simulink model "Robot_Model_Park"  (R2012b)
settings: Solver=ode45  StartTime=0.0  StopTime=T  FixedStep=dt  RelTol=1e-3
values from neighbouring files (symbols this model uses):
  bx = [0; 800; 800; 1600; 1600; 1600+L; 1600+L; 2400+L]    [TrajectoryCalc.m]
  by = [-dwall; -dwall; D-dwall; D-dwall; -dwall; -dwall; D-dwall; D-dwall]    [TrajectoryCalc.m]
  omega_park = [omega_park1; omega_park2; omega_park3]    [TrajectoryCalc.m]
  omegamax = 150*pi/180    (= 2.61799387799)    [TrajectoryCalc.m]
  psi0 = psi_park2(end)    [TrajectoryCalc.m]
  v_park = [v_park1; v_park2; v_park3]    [TrajectoryCalc.m]
  vmax = 500    [TrajectoryCalc.m]
  x0 = px_park2(end)    [TrajectoryCalc.m]
  y0 = py_park2(end)    [TrajectoryCalc.m]
settings Model: Creator=showe023  LastModifiedBy=Daniel
settings DataIOCC: SignalLoggingSaveFormat=ModelDataLogs
settings OptimizationCC: ExpressionDepthLimit=128
settings DebuggingCC: SolverPrmCheckMsg=none  MultiTaskDSMMsg=warning  MultiTaskCondExecSysMsg=none  StrictBusMsg=None
settings RTWCC: IncludeERTFirstTime=on
settings CodeAppCC: CustomSymbolStrType=$N$R$M_T  InternalIdentifier=Shortened

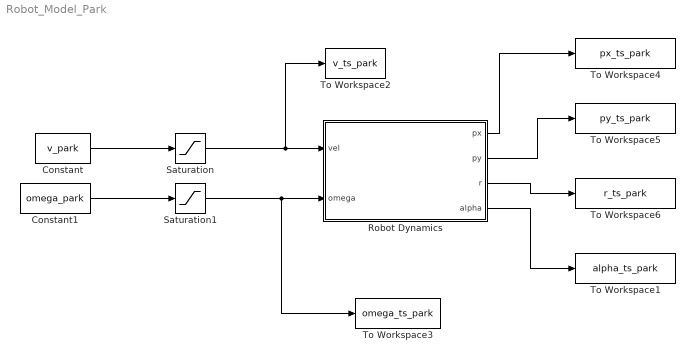
== system Robot_Model_Park ==
  Constant : Constant  Value=v_park
  Constant1 : Constant  Value=omega_park
  Robot Dynamics : Subsystem
  Saturation : Saturate  UpperLimit=vmax  LowerLimit=-vmax
  Saturation1 : Saturate  UpperLimit=omegamax  LowerLimit=-omegamax
  To Workspace1 : ToWorkspace  VariableName=alpha_ts_park  SampleTime=-1  SaveFormat=Timeseries
  To Workspace2 : ToWorkspace  VariableName=v_ts_park  SampleTime=-1  SaveFormat=Timeseries
  To Workspace3 : ToWorkspace  VariableName=omega_ts_park  SampleTime=-1  SaveFormat=Timeseries
  To Workspace4 : ToWorkspace  VariableName=px_ts_park  SampleTime=-1  SaveFormat=Timeseries
  To Workspace5 : ToWorkspace  VariableName=py_ts_park  SampleTime=-1  SaveFormat=Timeseries
  To Workspace6 : ToWorkspace  VariableName=r_ts_park  SampleTime=-1  SaveFormat=Timeseries
  wires:
  Robot Dynamics/1(px) -> To Workspace4/1
  Constant/1 -> Saturation/1
  Saturation/1 -> Robot Dynamics/1(vel), To Workspace2/1
  Robot Dynamics/2(py) -> To Workspace5/1
  Robot Dynamics/3(r) -> To Workspace6/1
  Robot Dynamics/4(alpha) -> To Workspace1/1
  Constant1/1 -> Saturation1/1
  Saturation1/1 -> To Workspace3/1, Robot Dynamics/2(omega)

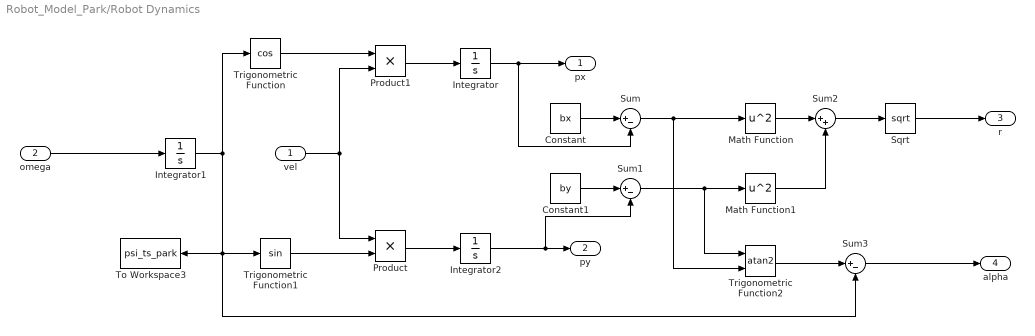
== system Robot_Model_Park/Robot Dynamics ==
  vel : Inport
  omega : Inport  Port=2
  Constant : Constant  Value=bx
  Constant1 : Constant  Value=by
  Integrator : Integrator  InitialCondition=x0
  Integrator1 : Integrator  InitialCondition=psi0
  Integrator2 : Integrator  InitialCondition=y0
  Math Function : Math  Operator=square  SaturateOnIntegerOverflow=on
  Math Function1 : Math  Operator=square  SaturateOnIntegerOverflow=on
  Product : Product
  Product1 : Product
  Sqrt : Sqrt  SaturateOnIntegerOverflow=on
  Sum : Sum  Inputs=|+-
  Sum1 : Sum  Inputs=|+-
  Sum2 : Sum  Inputs=|++
  Sum3 : Sum  Inputs=|+-
  To Workspace3 : ToWorkspace  VariableName=psi_ts_park  SampleTime=-1  SaveFormat=Timeseries
  Trigonometric Function : Trigonometry  Operator=cos
  Trigonometric Function1 : Trigonometry
  Trigonometric Function2 : Trigonometry  Operator=atan2
  px : Outport
  py : Outport  Port=2
  r : Outport  Port=3
  alpha : Outport  Port=4
  wires:
  omega/1 -> Integrator1/1
  Integrator1/1 -> Sum3/2, Trigonometric Function1/1, To Workspace3/1, Trigonometric Function/1
  Trigonometric Function/1 -> Product1/1
  Trigonometric Function1/1 -> Product/2
  Product/1 -> Integrator2/1
  Product1/1 -> Integrator/1
  Constant/1 -> Sum/1
  Sum/1 -> Trigonometric Function2/2, Math Function/1
  vel/1 -> Product/1, Product1/2
  Integrator/1 -> px/1, Sum/2
  Constant1/1 -> Sum1/1
  Integrator2/1 -> py/1, Sum1/2
  Math Function/1 -> Sum2/1
  Math Function1/1 -> Sum2/2
  Sum2/1 -> Sqrt/1
  Sqrt/1 -> r/1
  Sum1/1 -> Trigonometric Function2/1, Math Function1/1
  Trigonometric Function2/1 -> Sum3/1
  Sum3/1 -> alpha/1
